simulink model "shifter_matlab"  (R2022b)
settings: Solver=FixedStepDiscrete  StartTime=0.0  StopTime=30  FixedStep=0.05  RelTol=1e-3  EnableMultiTasking=on
PreLoadFcn:
  | % Input data
  | load shifter_data;
settings Model: Creator=jrivitus  LastModifiedBy=bensweet
settings SolverCC: AlgebraicLoopSolver=TrustRegion
settings DataIOCC: ExternalInput=[t, upThreshold, vehicleSpeed, downThreshold]  LimitDataPoints=on  LoadExternalInput=on  SaveFormat=Array  ReturnWorkspaceOutputs=off
settings OptimizationCC: ExpressionDepthLimit=2147483647  LifeSpan=inf
settings DebuggingCC: UnconnectedInputMsg=warning  UnconnectedOutputMsg=warning  UnconnectedLineMsg=warning  PregeneratedLibrarySubsystemCodeDiagnostic=none  SFMachineParentedDataDiag=warning
settings HardwareCC: ProdBitPerPointer=32  ProdBitPerSizeT=32  ProdBitPerPtrDiffT=32  ProdLargestAtomicFloat=None  ProdIntDivRoundTo=Undefined  ProdEndianess=Unspecified  ProdWordSize=32  ProdHWDeviceType=32-bit Generic
settings ModelReferenceCC: EnableRefExpFcnMdlSchedulingChecks=on  PropagateSignalLabelsOutOfModel=off
settings SFSimCC: SimUseLocalCustomCode=off
settings RTWCC: RTWUseLocalCustomCode=off  DLArmComputeVersion=19.05
settings CodeAppCC: StateflowObjectComments=on
settings GRTTargetCC: TargetLangStandard=C89/C90 (ANSI)  CombineOutputUpdateFcns=off  GRTInterface=on
settings ConfigComp: CovMetricSettings=dw  CovSaveCumulativeToWorkspaceVar=on  CovSaveSingleToWorkspaceVar=on  CovExternalEMLEnable=off  CovSFcnEnable=off

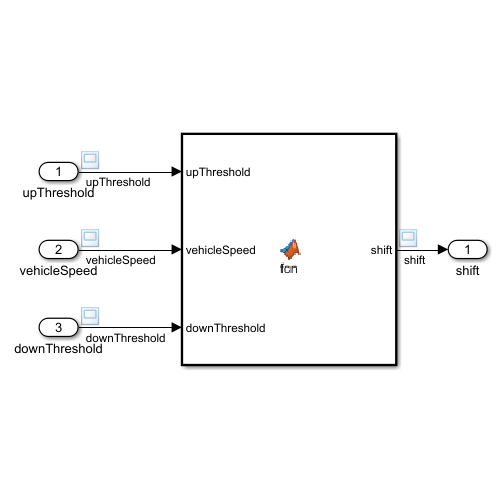
[thumbnail: Simulink's stored preview of the top-level diagram]
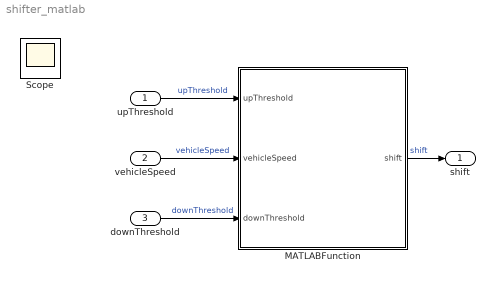
== system shifter_matlab ==
  upThreshold : Inport  OutDataTypeStr=double
  vehicleSpeed : Inport  Port=2  OutDataTypeStr=double
  downThreshold : Inport  Port=3  OutDataTypeStr=double
  MATLABFunction : MATLAB Function  TreatAsAtomicUnit=on
  shift : Outport  VectorParamsAs1DForOutWhenUnconnected=off
  Scope : Scope
  wires:
  MATLABFunction/1(shift) -> shift/1  "shift"
  upThreshold/1 -> MATLABFunction/1(upThreshold)  "upThreshold"
  vehicleSpeed/1 -> MATLABFunction/2(vehicleSpeed)  "vehicleSpeed"
  downThreshold/1 -> MATLABFunction/3(downThreshold)  "downThreshold"

== matlab function shifter_matlab/MATLABFunction ==
  data: upThreshold input; shift output; vehicleSpeed input; downThreshold input
function shift = fcn(upThreshold, vehicleSpeed, downThreshold)

if (vehicleSpeed > upThreshold)
    shift = 1;
elseif (vehicleSpeed < downThreshold)
    shift = -1;
else
    shift = 0;
end
